simulink model "Copy_of_CM13_2024a_MachE_for_UA_HIL"  (R2024a)
settings: Solver=ode1  StartTime=0.0  StopTime=Inf  FixedStep=0.001  RelTol=1e-3  EnableMultiTasking=on
PreLoadFcn:
  | % if ~length(which('cmcmd')), cmenv; end
PostLoadFcn:
  | if any(exist('dsrtsu_mdlpostloadfcn', 'file') ~= 0), dsrtsu_mdlpostloadfcn('Execute', bdroot); end
InitFcn:
  | , if any(exist('rtifpga_mdlclblib', 'file') ~= 0), rtifpga_mdlclblib('Init', bdroot); end,
  | , if any(exist('dsmpb_private', 'file') ~= 0), dsmpb_private('dsmpb_mdlclblib', 'Init', bdroot); end,
undefined symbols (not defined in the file or in its folder): AccelCmd, ActTqLF_Nm_, ActTqLR_Nm_, ActTqRF_Nm_, ActTqRR_Nm_, BattChargeLimitMaxPwr, BattChargeLimitSocBpts, BattChargeLimitTbl, BattChrgCapcty, BattDischargeLimitSocBpts, BattDischargeLimitTbl, BattDischargeMaxPwr, BattNumCellsParallel, BattNumCellsSeries, BattOpenVoltCapBpts, BattOpenVoltTbl, BattResistSocBpts, BattResistTbl, BattResistTempBpts, BrakeMaxPrs, BrakeMaxTrq, ChassisDistCg2FrontAxle, ChassisDistCg2RearAxle, ChassisVehMass, CltchCmd, CoastDown, DecelCmd, DiffRatio, DiscIntNeverNeededParam, EnvGravCnst, EnvPrs, EnvTemp, FuelSpecificGrav, GearCmd, h, InitStates, lgSw, limitedMCT, MCT, MtrEffSpdBpts, MtrEffTbl, MtrEffTrqBpts, MtrPwrMax, MtrTrqMax, planned_speed, planned_time, pMCT, RealSimPara, ref_speed, Ref_speed, ref_time, Ref_time, rticanmm_blockfcn, rticanmm_initfcn, SteeringCmd, SupvsryCtrlRegenBrkCutOffTbl, SupvsryCtrlRegenSpdBpts, TestScnrioCycleNum, US06, VEH
libraries: simulink x264, VSIGenLib x262, etargetslib x201, dsmpblib x161, CarMaker4SL x142, rtimmsu_dsrtlib x32, vehdynlibtire x24, autolibshared x19, vehdynlibsuspension x14, vehdynlibtirecommon x14, autolibutils x10, VsrLibWheel x8
(part 13 of 47)

== system Copy_of_CM13_2024a_MachE_for_UA_HIL/CarMaker/IPG Vehicle/Actuation and Outputs/MOOG Brake Actuator ==
  Brake Pedal command [%] : Inport
  " CAN Settings" : Subsystem
  BrakePedal Target Position Manual Bypass : Constant  Value=0
  BrakePedal TargetPosition Bypass Enable : Constant  Value=0
  Bus Selector : BusSelector  OutputSignals=ControlWord,TargetPositionFinal_cnt
  ControlWord bypass Enable : Constant  Value=0
  ControlWord bypass Override value : Constant  Value=0
  Data Type Conversion : DataTypeConversion  SaturateOnIntegerOverflow=off  RndMeth=Floor
  Data Type Conversion1 : DataTypeConversion  SaturateOnIntegerOverflow=off  RndMeth=Floor
  Data Type Conversion2 : DataTypeConversion  SaturateOnIntegerOverflow=off  RndMeth=Floor
  Gain : Gain
  Gain1 : Gain
  MOOG Interface : Subsystem
  RPDO3\ControlWord0\ISignal Value\ControlWord0 Value [BrakeAct_Config\Simulated ECUs\CANOpen_MOOG_02\Controller\TX\PDUs] : dsmpblib/Data Outport  Priority=-10000
      settings: SourceProductName=dSPACE Model Interface Package for Simulink (MIPS)
  RPDO3\ModesOfOperation\ISignal Value\ModesOfOperation Value [BrakeAct_Config\Simulated ECUs\CANOpen_MOOG_02\Controller\TX\PDUs] : dsmpblib/Data Outport  Priority=-10000
      settings: SourceProductName=dSPACE Model Interface Package for Simulink (MIPS)
  RPDO3\TargetPosition\ISignal Value\TargetPosition Value [BrakeAct_Config\Simulated ECUs\CANOpen_MOOG_02\Controller\TX\PDUs] : dsmpblib/Data Outport  Priority=-10000
      settings: SourceProductName=dSPACE Model Interface Package for Simulink (MIPS)
  Rate Limiter : RateLimiter  RisingSlewLimit=50  FallingSlewLimit=-50  SampleTimeMode=inherited
  Sine Wave : Sin  Amplitude=50  Bias=50  SampleTime=0
  Switch : Switch  Criteria=u2 > Threshold  SaturateOnIntegerOverflow=off  InputSameDT=off
  Switch1 : Switch  Criteria=u2 > Threshold  SaturateOnIntegerOverflow=off  InputSameDT=off
  Switch2 : Switch  Criteria=u2 > Threshold  SaturateOnIntegerOverflow=off  InputSameDT=off
  TPDO3\ActualPosition\ISignal Value\ActualPosition Value [BrakeAct_Config\Simulated ECUs\CANOpen_MOOG_02\Controller\RX\PDUs] : dsmpblib/Data Inport  Priority=10000
      settings: SourceProductName=dSPACE Model Interface Package for Simulink (MIPS)
  TPDO3\ModesOfOperationDisplay\ISignal Value\ModesOfOperationDisplay Value [BrakeAct_Config\Simulated ECUs\CANOpen_MOOG_02\Controller\RX\PDUs] : dsmpblib/Data Inport  Priority=10000
      settings: SourceProductName=dSPACE Model Interface Package for Simulink (MIPS)
  TPDO3\StatusWord0\ISignal Value\StatusWord0 Value [BrakeAct_Config\Simulated ECUs\CANOpen_MOOG_02\Controller\RX\PDUs] : dsmpblib/Data Inport  Priority=10000
      settings: SourceProductName=dSPACE Model Interface Package for Simulink (MIPS)
  Terminator : Terminator
  Terminator1 : Terminator
  Terminator2 : Terminator
  constant : Constant
  trace selection : Constant  Value=0
  wires:
  Switch/1 -> Switch2/1
  MOOG Interface/1(Commands) -> Bus Selector/1
  MOOG Interface/2(ActualPosition [pct]) -> Terminator/1  "BrakePedal_ActualPosition_pct"
  Bus Selector/2 -> Data Type Conversion2/1  "<TargetPositionFinal_cnt>"
  MOOG Interface/3(BrakeActuatorReady) -> Terminator1/1  "BrakeActuator_Ready_bool"
  Sine Wave/1 -> Switch/1
  Data Type Conversion2/1 -> RPDO3\TargetPosition\ISignal Value\TargetPosition Value [BrakeAct_Config\Simulated ECUs\CANOpen_MOOG_02\Controller\TX\PDUs]/1, Gain1/1  "TargetPosition_Cnt_Final"
  constant/1 -> Data Type Conversion/1
  BrakePedal TargetPosition Bypass Enable/1 -> Switch2/2
  trace selection/1 -> Switch/2
  TPDO3\ModesOfOperationDisplay\ISignal Value\ModesOfOperationDisplay Value [BrakeAct_Config\Simulated ECUs\CANOpen_MOOG_02\Controller\RX\PDUs]/1 -> MOOG Interface/5(Mode of operation in)  "Modes of operations"
  Data Type Conversion1/1 -> RPDO3\ControlWord0\ISignal Value\ControlWord0 Value [BrakeAct_Config\Simulated ECUs\CANOpen_MOOG_02\Controller\TX\PDUs]/1  "ControlWord_Final"
  Gain/1 -> MOOG Interface/2(TargetPosition [pct])  "BrakePedal_TargetlPosition_pct"
  Switch1/1 -> Data Type Conversion1/1
  TPDO3\ActualPosition\ISignal Value\ActualPosition Value [BrakeAct_Config\Simulated ECUs\CANOpen_MOOG_02\Controller\RX\PDUs]/1 -> MOOG Interface/4(ActualPosition_cnt in)  "ActualPosition_cnt"
  Bus Selector/1 -> Switch1/3  "<ControlWord>"
  ControlWord bypass Override value/1 -> Switch1/1
  TPDO3\StatusWord0\ISignal Value\StatusWord0 Value [BrakeAct_Config\Simulated ECUs\CANOpen_MOOG_02\Controller\RX\PDUs]/1 -> MOOG Interface/3(StatusWord in)  "StatusWord0"
  BrakePedal Target Position Manual Bypass/1 -> Rate Limiter/1
  ControlWord bypass Enable/1 -> Switch1/2
  Brake Pedal command [%]/1 -> Switch2/3
  " CAN Settings"/1(CAN_CommsOK_Flg) -> MOOG Interface/1(CAN_CommsOK_Flg)
  Gain1/1 -> Terminator2/1  "BrakePedal_CmdFinal_pct"
  Rate Limiter/1 -> Switch/3
  Switch2/1 -> Gain/1
  Data Type Conversion/1 -> RPDO3\ModesOfOperation\ISignal Value\ModesOfOperation Value [BrakeAct_Config\Simulated ECUs\CANOpen_MOOG_02\Controller\TX\PDUs]/1

== system Copy_of_CM13_2024a_MachE_for_UA_HIL/CarMaker/IPG Vehicle/Actuation and Outputs/Vehicle Accel Pedal Voltage Output ==
  note: Default value for MachE:
      | APP1_CmdFinal_V: 0.8016
      | APP2_CmdFinal_V: 0.4008
  APP_pct : Inport
  APP1Tbl : Lookup_n-D  NumberOfTableDimensions=1  BreakpointsForDimension1=[0 100]  Table=[16 78.8]  InternalRulePriority=Speed  RndMeth=Simplest
  APP2Tbl : Lookup_n-D  NumberOfTableDimensions=1  BreakpointsForDimension1=[0 100]  Table=[8 39.4]  InternalRulePriority=Speed  RndMeth=Simplest
  AccelPosition Bypass Enable : Constant  Value=0
  AccelPosition Manual Bypass [%] : Constant  Value=0
  Gain : Gain
  Gain1 : Gain
  Gain2 : Gain
  Gain3 : Gain  Gain=1/100
  Gain4 : Gain  Gain=1/100
  Product2 : Product
  Product3 : Product
  Rate Limiter : RateLimiter  RisingSlewLimit=50  FallingSlewLimit=-50  SampleTimeMode=inherited
  Switch2 : Switch  Criteria=u2 > Threshold  SaturateOnIntegerOverflow=off  InputSameDT=off
  TPS Channel 1 : dsmpblib/Data Outport  Priority=-10000
      settings: SourceProductName=dSPACE Model Interface Package for Simulink (MIPS)
  TPS Channel 2 : dsmpblib/Data Outport  Priority=-10000
      settings: SourceProductName=dSPACE Model Interface Package for Simulink (MIPS)
  Terminator2 : Terminator
  VRef : Constant  Value=5.01
  wires:
  Switch2/1 -> APP1Tbl/1, APP2Tbl/1, Gain2/1  "APP_CmdFinal_pct"
  APP_pct/1 -> Switch2/3
  AccelPosition Manual Bypass [%]/1 -> Rate Limiter/1
  AccelPosition Bypass Enable/1 -> Switch2/2
  Gain/1 -> TPS Channel 2/1  "APP2_CmdFinal_V"
  Gain1/1 -> TPS Channel 1/1  "APP1_CmdFinal_V"
  Gain2/1 -> Terminator2/1  "AccelPedal_CmdFinal_pct"
  Rate Limiter/1 -> Switch2/1
  VRef/1 -> Product2/2, Product3/1
  Gain4/1 -> Product3/2
  Product2/1 -> Gain1/1
  APP2Tbl/1 -> Gain4/1
  Gain3/1 -> Product2/1
  Product3/1 -> Gain/1
  APP1Tbl/1 -> Gain3/1

== system Copy_of_CM13_2024a_MachE_for_UA_HIL/CarMaker/IPG Vehicle/Brake/CreateBus Vhcl.Wheel.PT ==
  In : Inport
  BusCreator1 : BusCreator  Inputs=20
  Demux1 : Demux  Outputs=20
      settings: DisplayOption=none
  Out : Outport  VectorParamsAs1DForOutWhenUnconnected=off
  wires:
  Demux1/20 -> BusCreator1/20  "Vhcl Trq_DriveSrc_trg d3"
  Demux1/19 -> BusCreator1/19  "Vhcl Trq_DriveSrc_trg d2"
  Demux1/18 -> BusCreator1/18  "Vhcl Trq_DriveSrc_trg d1"
  Demux1/17 -> BusCreator1/17  "Vhcl Trq_DriveSrc_trg d0"
  Demux1/16 -> BusCreator1/16  "Vhcl Wheel RR WhlBearing"
  Demux1/15 -> BusCreator1/15  "Vhcl Wheel RR Trq_T2W"
  Demux1/14 -> BusCreator1/14  "Vhcl Wheel RR Trq_BrakeReg_trg"
  Demux1/13 -> BusCreator1/13  "Vhcl Wheel RR Trq_Brake"
  Demux1/12 -> BusCreator1/12  "Vhcl Wheel RL WhlBearing"
  Demux1/11 -> BusCreator1/11  "Vhcl Wheel RL Trq_T2W"
  Demux1/10 -> BusCreator1/10  "Vhcl Wheel RL Trq_BrakeReg_trg"
  Demux1/9 -> BusCreator1/9  "Vhcl Wheel RL Trq_Brake"
  Demux1/8 -> BusCreator1/8  "Vhcl Wheel FR WhlBearing"
  Demux1/7 -> BusCreator1/7  "Vhcl Wheel FR Trq_T2W"
  Demux1/6 -> BusCreator1/6  "Vhcl Wheel FR Trq_BrakeReg_trg"
  Demux1/5 -> BusCreator1/5  "Vhcl Wheel FR Trq_Brake"
  Demux1/4 -> BusCreator1/4  "Vhcl Wheel FL WhlBearing"
  Demux1/3 -> BusCreator1/3  "Vhcl Wheel FL Trq_T2W"
  Demux1/2 -> BusCreator1/2  "Vhcl Wheel FL Trq_BrakeReg_trg"
  Demux1/1 -> BusCreator1/1  "Vhcl Wheel FL Trq_Brake"
  BusCreator1/1 -> Out/1
  In/1 -> Demux1/1

== system Copy_of_CM13_2024a_MachE_for_UA_HIL/CarMaker/IPG Vehicle/CarAndTrailer/CarAndTrailerUpd ==
  Sync_In : Inport
  Vhcl.Steering : Inport  Port=2
  Vhcl.Motion : Inport  Port=3
  Vhcl.PoI : Inport  Port=4
  Vhcl.Wheel.FL : Inport  Port=5
  Vhcl.Wheel.FR : Inport  Port=6
  Vhcl.Wheel.RL : Inport  Port=7
  Vhcl.Wheel.RR : Inport  Port=8
  Car.Hitch.FrcTrq : Inport  Port=9
  Vhcl.Fr1A : Inport  Port=10
  CarAndTrailerUpd : S-Function  FunctionName=CM_Sfun  Parameters='CarAndTrUpd'  SFunctionDeploymentMode=off  EnableBusSupport=off
  CreateBus Brake.IF.In : Subsystem
  Sync_Out : Outport  VectorParamsAs1DForOutWhenUnconnected=off
  Brake.IF.In : Outport  Port=2  VectorParamsAs1DForOutWhenUnconnected=off
  wires:
  Vhcl.Fr1A/1 -> CarAndTrailerUpd/10  "user vehicle only"
  Vhcl.Steering/1 -> CarAndTrailerUpd/2
  Vhcl.Motion/1 -> CarAndTrailerUpd/3
  Vhcl.PoI/1 -> CarAndTrailerUpd/4
  Vhcl.Wheel.FL/1 -> CarAndTrailerUpd/5
  Vhcl.Wheel.FR/1 -> CarAndTrailerUpd/6
  Car.Hitch.FrcTrq/1 -> CarAndTrailerUpd/9
  Vhcl.Wheel.RR/1 -> CarAndTrailerUpd/8
  Vhcl.Wheel.RL/1 -> CarAndTrailerUpd/7
  CarAndTrailerUpd/2 -> CreateBus Brake.IF.In/1(In)
  CreateBus Brake.IF.In/1(Out) -> Brake.IF.In/1
  CarAndTrailerUpd/1 -> Sync_Out/1
  Sync_In/1 -> CarAndTrailerUpd/1

== system Copy_of_CM13_2024a_MachE_for_UA_HIL/CarMaker/IPG Vehicle/CarAndTrailer/Forces ==
  Sync_In : Inport
  TireFL_In : Inport  Port=2
  TireFR_In : Inport  Port=3
  TireRL_In : Inport  Port=4
  TireRR_In : Inport  Port=5
  lSpring : Inport  Port=6
  vDamp : Inport  Port=7
  lStabi : Inport  Port=8
  lBuf : Inport  Port=9
  External Suspension Forces : Subsystem
  Suspension Forces : Subsystem
  Tires : Subsystem
  Vehicle Forces : Subsystem
  Sync_Out : Outport  VectorParamsAs1DForOutWhenUnconnected=off
  Car.Virtual : Outport  Port=2  VectorParamsAs1DForOutWhenUnconnected=off
  Car.Aero : Outport  Port=3  VectorParamsAs1DForOutWhenUnconnected=off
  Car.Load : Outport  Port=4  VectorParamsAs1DForOutWhenUnconnected=off
  TireFL_Out : Outport  Port=5  VectorParamsAs1DForOutWhenUnconnected=off
  TireFR_Out : Outport  Port=6  VectorParamsAs1DForOutWhenUnconnected=off
  TireRL_Out : Outport  Port=7  VectorParamsAs1DForOutWhenUnconnected=off
  TireRR_Out : Outport  Port=8  VectorParamsAs1DForOutWhenUnconnected=off
  FSpring_ext : Outport  Port=9  VectorParamsAs1DForOutWhenUnconnected=off
  FDamp_ext : Outport  Port=10  VectorParamsAs1DForOutWhenUnconnected=off
  FStabi_ext : Outport  Port=11  VectorParamsAs1DForOutWhenUnconnected=off
  FBuf_ext : Outport  Port=12  VectorParamsAs1DForOutWhenUnconnected=off
  wires:
  lBuf/1 -> External Suspension Forces/5(lBuf), Suspension Forces/5(lBuf)
  lStabi/1 -> External Suspension Forces/4(lStabi), Suspension Forces/4(lStabi)
  vDamp/1 -> External Suspension Forces/3(vDamp), Suspension Forces/3(vDamp)
  Tires/4(TireRR_Out) -> TireRR_Out/1
  Tires/3(TireRL_Out) -> TireRL_Out/1
  Tires/2(TireFR_Out) -> TireFR_Out/1
  Tires/1(TireFL_Out) -> TireFL_Out/1
  TireRR_In/1 -> Tires/5(TireRR_In)
  TireRL_In/1 -> Tires/4(TireRL_In)
  TireFR_In/1 -> Tires/3(TireFR_In)
  TireFL_In/1 -> Tires/2(TireFL_In)
  External Suspension Forces/4(FBuf_ext) -> FBuf_ext/1
  Sync_In/1 -> External Suspension Forces/1(Sync_In), Tires/1(Sync_In), Vehicle Forces/1(Sync_In)
  Vehicle Forces/1(Sync_Out) -> Suspension Forces/1(Sync_In)
  Vehicle Forces/2(Car.Virtual) -> Car.Virtual/1
  Vehicle Forces/3(Car.Aero) -> Car.Aero/1
  Vehicle Forces/4(Car.Load) -> Car.Load/1
  lSpring/1 -> External Suspension Forces/2(lSpring), Suspension Forces/2(lSpring)
  External Suspension Forces/2(FDamp_ext) -> FDamp_ext/1
  External Suspension Forces/3(FStabi_ext) -> FStabi_ext/1
  External Suspension Forces/1(FSpring_ext) -> FSpring_ext/1
  Suspension Forces/1(Sync_Out) -> Sync_Out/1

== system Copy_of_CM13_2024a_MachE_for_UA_HIL/CarMaker/IPG Vehicle/CarAndTrailer/Kinematics ==
  Sync_In : Inport
  Steer.IF : Inport  Port=2
  Kinematics : S-Function  FunctionName=CM_Sfun  Parameters='Kinematics'  SFunctionDeploymentMode=off  EnableBusSupport=off
  Sync_Out : Outport  VectorParamsAs1DForOutWhenUnconnected=off
  TireFL_In : Outport  Port=2  VectorParamsAs1DForOutWhenUnconnected=off
  TireFR_In : Outport  Port=3  VectorParamsAs1DForOutWhenUnconnected=off
  TireRL_In : Outport  Port=4  VectorParamsAs1DForOutWhenUnconnected=off
  TireRR_In : Outport  Port=5  VectorParamsAs1DForOutWhenUnconnected=off
  lSpring : Outport  Port=6  VectorParamsAs1DForOutWhenUnconnected=off
  vDamp : Outport  Port=7  VectorParamsAs1DForOutWhenUnconnected=off
  lStabi : Outport  Port=8  VectorParamsAs1DForOutWhenUnconnected=off
  lBuf : Outport  Port=9  VectorParamsAs1DForOutWhenUnconnected=off
  wires:
  Kinematics/9 -> lBuf/1
  Kinematics/8 -> lStabi/1
  Kinematics/2 -> TireFL_In/1
  Kinematics/3 -> TireFR_In/1
  Kinematics/4 -> TireRL_In/1
  Kinematics/5 -> TireRR_In/1
  Kinematics/6 -> lSpring/1
  Kinematics/7 -> vDamp/1
  Sync_In/1 -> Kinematics/1
  Kinematics/1 -> Sync_Out/1
  Steer.IF/1 -> Kinematics/2

== system Copy_of_CM13_2024a_MachE_for_UA_HIL/CarMaker/IPG Vehicle/CarAndTrailer/Kinetics ==
  Sync_In : Inport
  Car.Virtual : Inport  Port=2
  Car.Aero : Inport  Port=3
  Car.Load : Inport  Port=4
  TireFL.Out : Inport  Port=5
  TireFR.Out : Inport  Port=6
  TireRL.Out : Inport  Port=7
  TireRR.Out : Inport  Port=8
  FSpring_ext : Inport  Port=9
  FDamp_ext : Inport  Port=10
  FStabi_ext : Inport  Port=11
  FBuf_ext : Inport  Port=12
  Bus Creator : BusCreator  Inputs=4
  Bus Creator1 : BusCreator  Inputs=12
  Bus Creator2 : BusCreator  Inputs=6
  Bus Creator3 : BusCreator  Inputs=6
  Bus Creator4 : BusCreator  Inputs=4
  Demux : Demux  Outputs=12
      settings: DisplayOption=none
  Demux1 : Demux  Outputs=6
      settings: DisplayOption=none
  Demux2 : Demux  Outputs=6
      settings: DisplayOption=none
  Demux3 : Demux
      settings: DisplayOption=none
  Demux4 : Demux
      settings: DisplayOption=none
  Kinetics : S-Function  FunctionName=CM_Sfun  Parameters='Kinetics'  SFunctionDeploymentMode=off  EnableBusSupport=off
  Sync_Out : Outport  VectorParamsAs1DForOutWhenUnconnected=off
  Trailer.Load : Outport  Port=2  VectorParamsAs1DForOutWhenUnconnected=off
  Car.Hitch : Outport  Port=3  VectorParamsAs1DForOutWhenUnconnected=off
  Car.Fr1 : Outport  Port=4  VectorParamsAs1DForOutWhenUnconnected=off
  Car.Trq_T2W : Outport  Port=5  VectorParamsAs1DForOutWhenUnconnected=off
  WheelCarrier.Misc : Outport  Port=6  VectorParamsAs1DForOutWhenUnconnected=off
  wires:
  FBuf_ext/1 -> Kinetics/12
  Sync_In/1 -> Kinetics/1
  Kinetics/1 -> Sync_Out/1
  Car.Aero/1 -> Kinetics/3
  Car.Virtual/1 -> Kinetics/2
  Bus Creator1/1 -> Trailer.Load/1
  Demux/1 -> Bus Creator1/1  "Trailer Load_0 mass"
  Demux/2 -> Bus Creator1/2  "Trailer Load_0 tx"
  Demux/3 -> Bus Creator1/3  "Trailer Load_0 ty"
  Demux/4 -> Bus Creator1/4  "Trailer Load_0 tz"
  Kinetics/2 -> Demux/1
  Demux/5 -> Bus Creator1/5  "Trailer Load_1 mass"
  Demux/6 -> Bus Creator1/6  "Trailer Load_1 tx"
  Demux/7 -> Bus Creator1/7  "Trailer Load_1 ty"
  Demux/8 -> Bus Creator1/8  "Trailer Load_1 tz"
  Demux/9 -> Bus Creator1/9  "Trailer Load_2 mass"
  Demux/10 -> Bus Creator1/10  "Trailer Load_2 tx"
  Demux/11 -> Bus Creator1/11  "Trailer Load_2 ty"
  Demux/12 -> Bus Creator1/12  "Trailer Load_2 tz"
  Demux1/1 -> Bus Creator2/1  "Car Hitch tx"
  Demux1/2 -> Bus Creator2/2  "Car Hitch ty"
  Demux1/3 -> Bus Creator2/3  "Car Hitch tz"
  Demux1/4 -> Bus Creator2/4  "Car Hitch vx"
  Demux1/5 -> Bus Creator2/5  "Car Hitch vy"
  Demux1/6 -> Bus Creator2/6  "Car Hitch vz"
  Kinetics/3 -> Demux1/1
  Bus Creator2/1 -> Car.Hitch/1
  Demux2/1 -> Bus Creator3/1  "Car Fr1 rx"
  Demux2/2 -> Bus Creator3/2  "Car Fr1 ry"
  Demux2/3 -> Bus Creator3/3  "Car Fr1 rz"
  Demux2/4 -> Bus Creator3/4  "Car Fr1 rvx"
  Demux2/5 -> Bus Creator3/5  "Car Fr1 rvy"
  Demux2/6 -> Bus Creator3/6  "Car Fr1 rvz"
  Bus Creator3/1 -> Car.Fr1/1
  Kinetics/4 -> Demux2/1
  Car.Load/1 -> Kinetics/4
  Demux3/1 -> Bus Creator4/1  "car Susp FL GenInert2"
  Demux3/2 -> Bus Creator4/2  "car Susp FR GenInert2"
  Demux3/3 -> Bus Creator4/3  "car Susp FL GenFrc2"
  Demux3/4 -> Bus Creator4/4  "car Susp FR GenFrc2"
  Bus Creator4/1 -> WheelCarrier.Misc/1
  Bus Creator/1 -> Car.Trq_T2W/1
  Demux4/4 -> Bus Creator/4  "Car Trq_T2WRR"
  Demux4/3 -> Bus Creator/3  "Car Trq_T2WRL"
  Demux4/2 -> Bus Creator/2  "Car Trq_T2WFR"
  Demux4/1 -> Bus Creator/1  "Car Trq_T2WFL"
  TireFL.Out/1 -> Kinetics/5
  TireFR.Out/1 -> Kinetics/6
  TireRL.Out/1 -> Kinetics/7
  TireRR.Out/1 -> Kinetics/8
  FSpring_ext/1 -> Kinetics/9
  FDamp_ext/1 -> Kinetics/10
  FStabi_ext/1 -> Kinetics/11
  Kinetics/6 -> Demux3/1
  Kinetics/5 -> Demux4/1

== system Copy_of_CM13_2024a_MachE_for_UA_HIL/CarMaker/IPG Vehicle/CarAndTrailer/Steering ==
  note: When replacing the entire steering system,
      | be sure to disable the IPG steering model by using the steering
      | model 'Model Manager off' in the vehicle GUI.
  Sync_In : Inport
  VhclCtrl.Steering : Inport  Port=2
  Bus Creator1 : BusCreator  Inputs=16
  Bus Creator2 : BusCreator  Inputs=5
  Demux : Demux  Outputs=21
      settings: DisplayOption=none
  Steering : S-Function  FunctionName=CM_Sfun  Parameters='Steering'  SFunctionDeploymentMode=off  EnableBusSupport=off
  Terminator : Terminator
  Sync_Out : Outport  VectorParamsAs1DForOutWhenUnconnected=off
  Steer.IF : Outport  Port=2  VectorParamsAs1DForOutWhenUnconnected=off
  wires:
  Demux/21 -> Bus Creator2/5  "Steering IF R Inert"
  Demux/20 -> Bus Creator2/4  "Steering IF R Frc"
  Demux/19 -> Bus Creator2/3  "Steering IF L Inert"
  Demux/18 -> Bus Creator2/2  "Steering IF L Frc"
  Demux/17 -> Bus Creator2/1  "Steering IF SteerByTrq"
  Demux/16 -> Bus Creator1/16  "Steering IF R iSteer2q"
  Demux/15 -> Bus Creator1/15  "Steering IF R qpp"
  Demux/14 -> Bus Creator1/14  "Steering IF R qp"
  Demux/13 -> Bus Creator1/13  "Steering IF R q"
  Demux/12 -> Bus Creator1/12  "Steering IF L iSteer2q"
  Demux/11 -> Bus Creator1/11  "Steering IF L qpp"
  Demux/10 -> Bus Creator1/10  "Steering IF L qp"
  Demux/9 -> Bus Creator1/9  "Steering IF L q"
  Demux/8 -> Bus Creator1/8  "Steering IF AssistTrqPin"
  Demux/7 -> Bus Creator1/7  "Steering IF AssistTrqCol"
  Demux/6 -> Bus Creator1/6  "Steering IF AssistFrc"
  Demux/5 -> Bus Creator1/5  "Steering IF TrqStatic"
  Demux/4 -> Bus Creator1/4  "Steering IF Trq"
  Demux/3 -> Bus Creator1/3  "Steering IF AngAcc"
  Demux/2 -> Bus Creator1/2  "Steering IF AngVel"
  Demux/1 -> Bus Creator1/1  "Steering IF Ang"
  Bus Creator1/1 -> Steer.IF/1
  Steering/2 -> Demux/1
  Bus Creator2/1 -> Terminator/1  "Steer IF (in)"
  VhclCtrl.Steering/1 -> Steering/2
  Steering/1 -> Sync_Out/1
  Sync_In/1 -> Steering/1

== system Copy_of_CM13_2024a_MachE_for_UA_HIL/CarMaker/IPG Vehicle/CarAndTrailer/Trailer ==
  Sync_In : Inport
  Trailer.Load : Inport  Port=2
  Car.Hitch : Inport  Port=3
  Car.Fr1 : Inport  Port=4
  Car.Trq_T2W : Inport  Port=5
  WheelCarrier.Misc : Inport  Port=6
  CreateBus Car.Hitch.FrcTrq : Subsystem
  CreateBus Vhcl.Motion : Subsystem
  CreateBus Vhcl.PoI : Subsystem
  CreateBus Vhcl.Steering : Subsystem
  CreateBus Vhcl.Wheel.FL : Subsystem
  CreateBus Vhcl.Wheel.FR : Subsystem
  CreateBus Vhcl.Wheel.RL : Subsystem
  CreateBus Vhcl.Wheel.RR : Subsystem
  Trailer : S-Function  FunctionName=CM_Sfun  Parameters='Trailer'  SFunctionDeploymentMode=off  EnableBusSupport=off
  Sync_Out : Outport  VectorParamsAs1DForOutWhenUnconnected=off
  Vhcl.Steering : Outport  Port=2  VectorParamsAs1DForOutWhenUnconnected=off
  Vhcl.Motion : Outport  Port=3  VectorParamsAs1DForOutWhenUnconnected=off
  Vhcl.PoI : Outport  Port=4  VectorParamsAs1DForOutWhenUnconnected=off
  Vhcl.Wheel.FL : Outport  Port=5  VectorParamsAs1DForOutWhenUnconnected=off
  Vhcl.Wheel.FR : Outport  Port=6  VectorParamsAs1DForOutWhenUnconnected=off
  Vhcl.Wheel.RL : Outport  Port=7  VectorParamsAs1DForOutWhenUnconnected=off
  Vhcl.Wheel.RR : Outport  Port=8  VectorParamsAs1DForOutWhenUnconnected=off
  Car.Hitch.FrcTrq : Outport  Port=9  VectorParamsAs1DForOutWhenUnconnected=off
  wires:
  Trailer/2 -> CreateBus Vhcl.Steering/1(In1)
  CreateBus Vhcl.Steering/1(Out1) -> Vhcl.Steering/1  "Vhcl.Steering"
  Trailer/3 -> CreateBus Vhcl.Motion/1(In1)
  Trailer/4 -> CreateBus Vhcl.PoI/1(In1)
  Trailer/5 -> CreateBus Vhcl.Wheel.FL/1(In1)
  Trailer/6 -> CreateBus Vhcl.Wheel.FR/1(In1)
  Trailer/7 -> CreateBus Vhcl.Wheel.RL/1(In1)
  Trailer/9 -> CreateBus Car.Hitch.FrcTrq/1(In1)
  Trailer/8 -> CreateBus Vhcl.Wheel.RR/1(In1)
  CreateBus Vhcl.Wheel.RR/1(Out1) -> Vhcl.Wheel.RR/1  "Vhcl.Wheel.RR"
  CreateBus Vhcl.Wheel.RL/1(Out1) -> Vhcl.Wheel.RL/1  "Vhcl.Wheel.RL"
  CreateBus Vhcl.Wheel.FR/1(Out1) -> Vhcl.Wheel.FR/1  "Vhcl.Wheel.FR"
  CreateBus Vhcl.Wheel.FL/1(Out1) -> Vhcl.Wheel.FL/1  "Vhcl.Wheel.FL"
  CreateBus Vhcl.PoI/1(Out1) -> Vhcl.PoI/1  "Vhcl.PoI"
  CreateBus Vhcl.Motion/1(Out1) -> Vhcl.Motion/1  "Vhcl.Motion"
  Car.Trq_T2W/1 -> Trailer/5
  WheelCarrier.Misc/1 -> Trailer/6
  CreateBus Car.Hitch.FrcTrq/1(Out1) -> Car.Hitch.FrcTrq/1  "Car.Hitch.FrcTrq"
  Car.Fr1/1 -> Trailer/4
  Car.Hitch/1 -> Trailer/3
  Trailer.Load/1 -> Trailer/2
  Trailer/1 -> Sync_Out/1
  Sync_In/1 -> Trailer/1

== system Copy_of_CM13_2024a_MachE_for_UA_HIL/CarMaker/IPG Vehicle/Driver and Drive Cycle/Automation_Spd_selection ==
  note: Auther@MaxChen
  note: Note: Since all v_vut is assinged to init velocity,
      | we will use this number as the target testrun speed
  note: If CM reach postprocessing,
      | or vehicle has driven more than 150meter, set speed to 0
  note: TODO: This delay need to be larger. Maybe a real-time of 5 seconds
  note: If AEB flag is triggered, set speed to 0
      | If AEB flag is cleared:
      | 	if Master SW is ON, use TestRun File Speed Demond
      | 	else speed is 0
  AEB_IS_Triggered : Inport
  A_M_SW_sig : Inport  Port=2
  0_speed : Constant  Value=0
  Compare To Constant : simulink/Logic and Bit Operations/Compare To Constant  relop===  const=10  OutDataTypeStr=boolean
  Compare To Constant1 : simulink/Logic and Bit Operations/Compare To Constant  relop=>=  const=150  OutDataTypeStr=boolean
  Delay : Delay  DelayLength=5
  OR : Logic  Operator=OR  IconShape=distinctive  AllPortsSameDT=off  OutDataTypeStr=boolean
  Read CM Dict11 : CarMaker4SL/Read CM Dict  xname=Vhcl.Distance  xsync=off  xstime=Continuous
  Read CM Dict7 : CarMaker4SL/Read CM Dict  xname=SC.State  xsync=off  xstime=Continuous
  Read CM Parameter : CarMaker4SL/Read CM Parameter  xfile=Testrun  xkey=DrivMan.Init.Velocity  xnout=1  xdefaults=0  xmuxed=on  xstime=Continuous
      settings: SourceProductName=CarMaker4SL
  Switch : Switch  Criteria=u2 > Threshold  SaturateOnIntegerOverflow=off  InputSameDT=off
  Switch1 : Switch  Criteria=u2 > Threshold  SaturateOnIntegerOverflow=off  InputSameDT=off
  Switch2 : Switch  Criteria=u2 > Threshold  SaturateOnIntegerOverflow=off  InputSameDT=off
  Spd : Outport
  wires:
  AEB_IS_Triggered/1 -> Switch/2
  Switch/1 -> Switch2/3
  A_M_SW_sig/1 -> Delay/1
  0_speed/1 -> Switch1/3, Switch/1, Switch2/1
  Switch1/1 -> Switch/3
  Delay/1 -> Switch1/2
  Read CM Dict7/1 -> Compare To Constant/1  "SC.State"
  Compare To Constant/1 -> OR/2
  Switch2/1 -> Spd/1
  Read CM Parameter/1 -> Switch1/1  "v_vut"
  Read CM Dict11/1 -> Compare To Constant1/1  "Vhcl.Distance"
  Compare To Constant1/1 -> OR/1
  OR/1 -> Switch2/2

== system Copy_of_CM13_2024a_MachE_for_UA_HIL/CarMaker/IPG Vehicle/Driver and Drive Cycle/Driver and PI with FF Control ==
  Vehicle_Spd_kph : Inport
  Vehicle_SpdDmd_kph : Inport  Port=2
  Bus Creator : BusCreator  Inputs=6
  Constant : Constant
  Memory1 : Memory
  Memory2 : Memory
  SpdSat : Saturate  UpperLimit=190  LowerLimit=-5
  Vehicle Speed Controller : Subsystem
  km to miles : Gain  Gain=1/1.609344
  DriverBus : Outport
  wires:
  Vehicle Speed Controller/1(AcceleratorPedalPos) -> Bus Creator/2  "AccelPedalCmd"
  Vehicle_SpdDmd_kph/1 -> Memory1/1
  Constant/1 -> Bus Creator/1  "Drive"
  Vehicle Speed Controller/3(BrakeSwitch) -> Bus Creator/4
  SpdSat/1 -> Vehicle Speed Controller/1(RefSpd), km to miles/1, Bus Creator/5  "RefSpd [km/hr]"
  Vehicle Speed Controller/2(BrakePedalPos) -> Bus Creator/3  "BrakePedalCmd"
  Bus Creator/1 -> DriverBus/1  "DriverBus"
  Vehicle_Spd_kph/1 -> Memory2/1
  km to miles/1 -> Bus Creator/6  "RefSpd [mph]"
  Memory1/1 -> SpdSat/1
  Memory2/1 -> Vehicle Speed Controller/2(VehicleSpeed)

== system Copy_of_CM13_2024a_MachE_for_UA_HIL/CarMaker/IPG Vehicle/Driver and Drive Cycle/Get Cycle Clock Time ==
  Cycle Trigger : Inport
  Add1 : Sum  Inputs=+-
  Clock1 : Clock
  Clock2 : Clock
  Data Type Conversion : DataTypeConversion  OutDataTypeStr=double  SaturateOnIntegerOverflow=off  RndMeth=Floor
  Memory4 : Memory
  Switch : Switch  Criteria=u2 > Threshold  SaturateOnIntegerOverflow=off  InputSameDT=off
  tCycle : Outport
  wires:
  Switch/1 -> Add1/2, Memory4/1
  Clock1/1 -> Add1/1
  Clock2/1 -> Switch/3
  Add1/1 -> tCycle/1  "tCycle"
  Memory4/1 -> Switch/1
  Cycle Trigger/1 -> Data Type Conversion/1
  Data Type Conversion/1 -> Switch/2

== system Copy_of_CM13_2024a_MachE_for_UA_HIL/CarMaker/IPG Vehicle/Driver and Drive Cycle/IDM ==
  note: In IPG, when the ego vehicle slipped side to side, it will ignore the front vehicle as in the path. The <RadarL> "detects nearest point in the path" , thus ego vehilce will no longer consider the front vehilce as "in path" and ACC/IDM will have incorrect output.
      |
      | Second object sensor <Backup> is added, it dectects nearest point, ensuring ego vehicle stopped at close range.
  CM_Time : Inport
  Add1 : Sum
  Add2 : Sum
  Add3 : Sum  Commented=on
  Bus Selector : BusSelector  OutputSignals=NearPnt ds x,NearPnt ds y,NearPnt dv x
  Bus Selector1 : BusSelector  OutputSignals=dtct
  Bus Selector2 : BusSelector  OutputSignals=dtct
  Bus Selector3 : BusSelector  OutputSignals=NearPnt ds x,NearPnt ds y
  Bus Selector4 : BusSelector  Commented=on  OutputSignals=NearPnt ds x,NearPnt ds y,NearPnt dv x
  Bus Selector5 : BusSelector  Commented=on  OutputSignals=dtct
  Bus Selector6 : BusSelector  OutputSignals=Dist,Vrel
  Compare To Constant : simulink/Logic and Bit Operations/Compare To Constant  relop=>=  const=30  OutDataTypeStr=boolean
  Constant : Constant  Value=0
  Constant1 : Constant  Value=99999
  Constant2 : Constant  Value=99999
  Dis2lead_Raw : Scope
  Math Function{,1..3} (4 alike) : Math  Operator=square
  Math Function4 : Math  Commented=on  Operator=square
  Math Function5 : Math  Commented=on  Operator=square
  ObjIndex : Scope
  Object Sensor 1 : CarMaker4SL/Sensors/Object Sensor  xname=RadarS  xstime=Continuous
      settings: SourceProductName=CarMaker4SL
  Object Sensor 2 : CarMaker4SL/Sensors/Object Sensor  xname=RadarL  xstime=Continuous
      settings: SourceProductName=CarMaker4SL
  Object Sensor Object : CarMaker4SL/Sensors/Object Sensor Object  Commented=on  xname=RadarL  ximode=Observed Objects  xstime=Continuous
      settings: SourceProductName=CarMaker4SL
  Object Sensor Object 1 : CarMaker4SL/Sensors/Object Sensor Object  xname=INPORT  ximode=Observed Objects  xstime=Continuous
      settings: SourceProductName=CarMaker4SL
  Object Sensor Object 2 : CarMaker4SL/Sensors/Object Sensor Object  xname=INPORT  ximode=Observed Objects  xstime=Continuous
      settings: SourceProductName=CarMaker4SL
  Radar Sensor : CarMaker4SL/Sensors/Radar Sensor  xname=RadarReal  xstime=Continuous
      settings: SourceProductName=CarMaker4SL
  Radar Sensor Object : CarMaker4SL/Sensors/Radar Sensor Object  xname=INPORT  ximode=Observed Objects  xstime=Continuous
      settings: SourceProductName=CarMaker4SL
  Read CM Dict1 : CarMaker4SL/Read CM Dict  xname=Car.v  xsync=off  xstime=Continuous
  Scope1 : Scope  Commented=on
  Scope2 : Scope  Commented=on
  Scope3 : Scope
  Scope4 : Scope
  Square Root : Sqrt
  Square Root1 : Sqrt
  Square Root2 : Sqrt  Commented=on
  Subsystem : Subsystem
  Switch1 : Switch  Criteria=u2 > Threshold  SaturateOnIntegerOverflow=off  InputSameDT=off
  ego_ref_spd_m/s : Outport
  wires:
  Add1/1 -> Square Root/1
  Bus Selector1/1 -> Subsystem/1(is_detected)  "<dtct>"
  Bus Selector/3 -> Subsystem/4(rel_front_spd_m/s)  "<NearPnt dv x>"
  Object Sensor Object 2/3 -> Bus Selector1/1
  Read CM Dict1/1 -> Subsystem/2(ego_spd_m/s)  "VehSpd"
  Math Function/1 -> Add1/1
  Object Sensor Object 2/5 -> Bus Selector/1
  Math Function1/1 -> Add1/2
  Object Sensor 2/1 -> Object Sensor Object 2/1
  Constant2/1 -> Object Sensor Object 2/2
  Bus Selector/1 -> Math Function/1  "<NearPnt ds x>"
  Bus Selector/2 -> Math Function1/1  "<NearPnt ds y>"
  Subsystem/1(ego_ref_spd_m/s) -> Switch1/1
  Object Sensor 1/1 -> Object Sensor Object 1/1
  Constant1/1 -> Object Sensor Object 1/2
  Object Sensor Object 1/3 -> Bus Selector2/1
  Bus Selector2/1 -> Subsystem/5(backup_detected)  "<dtct>"
  CM_Time/1 -> [CM_Time]
  Compare To Constant/1 -> Switch1/2
  Constant/1 -> Switch1/3
  Switch1/1 -> ego_ref_spd_m/s/1
  [CM_Time] -> Compare To Constant/1
  Object Sensor Object 1/5 -> Bus Selector3/1
  Math Function3/1 -> Add2/2
  Math Function2/1 -> Add2/1
  Add2/1 -> Square Root1/1
  Bus Selector3/1 -> Math Function2/1  "<NearPnt ds x>"
  Bus Selector3/2 -> Math Function3/1  "<NearPnt ds y>"
  Bus Selector4/2 -> Math Function5/1  "<NearPnt ds y>"
  Bus Selector4/1 -> Math Function4/1  "<NearPnt ds x>"
  Object Sensor Object/3 -> Bus Selector5/1
  Object Sensor Object/5 -> Bus Selector4/1
  Square Root2/1 -> Scope1/1
  Bus Selector4/3 -> Scope2/1  "<NearPnt dv x>"
  Add3/1 -> Square Root2/1
  Math Function4/1 -> Add3/1
  Math Function5/1 -> Add3/2
  Square Root1/1 -> Subsystem/6(front_obj_dist_m)
  Square Root/1 -> Subsystem/3(int_veh_dist_m), Dis2lead_Raw/1
  Radar Sensor/1 -> Radar Sensor Object/1
  Radar Sensor Object/2 -> Bus Selector6/1
  Bus Selector6/1 -> Scope3/1  "<Dist>"
  Bus Selector6/2 -> Scope4/1  "<Vrel>"
  Object Sensor Object 2/1 -> ObjIndex/1

== system Copy_of_CM13_2024a_MachE_for_UA_HIL/CarMaker/IPG Vehicle/Mach-E CAN BM/Subsystem ==
  note: softRCM ECU
  Bus Creator : BusCreator  Inputs=5
  Logic : Subsystem
  Noise Generators : Subsystem  Commented=on
  Read CM Dict : CarMaker4SL/Read CM Dict  xname=Car.RollVel  xsync=off  xstime=Continuous
  Read CM Dict1 : CarMaker4SL/Read CM Dict  xname=Car.YawRate  xsync=off  xstime=Continuous
  Read CM Dict2 : CarMaker4SL/Read CM Dict  xname=Car.ax  xsync=off  xstime=Continuous
  Read CM Dict3 : CarMaker4SL/Read CM Dict  xname=Car.ay  xsync=off  xstime=Continuous
  Read CM Dict4 : CarMaker4SL/Read CM Dict  xname=Car.az  xsync=off  xstime=Continuous
  AccelYaw_out : Outport
  wires:
  Logic/1(Out1) -> AccelYaw_out/1
  Bus Creator/1 -> Logic/1(In1)
  Read CM Dict4/1 -> Bus Creator/5  "a_z_Vehicle_CoG_withG[m|s2]"
  Read CM Dict3/1 -> Bus Creator/4  "a_y_Vehicle_CoG_withG[m|s2]"
  Read CM Dict2/1 -> Bus Creator/3  "a_x_Vehicle_CoG_withG[m|s2]"
  Read CM Dict/1 -> Bus Creator/1  "RollRate_Vehicle_CoG[rad|s]"
  Read CM Dict1/1 -> Bus Creator/2  "YawRate_Vehicle_CoG[rad|s]"

== system Copy_of_CM13_2024a_MachE_for_UA_HIL/CarMaker/IPG Vehicle/Mach-E CAN BM/Subsystem1 ==
  note: softRCM ECU
  Roll : Inport
  Yaw : Inport  Port=2
  A_x : Inport  Port=3
  A_y : Inport  Port=4
  A_z : Inport  Port=5
  Add{,1..4} (5 alike) : Sum
  Bus Creator : BusCreator  Inputs=5
  Logic : Subsystem
  Noise Generators : Subsystem  Commented=on
  Read CM Dict : CarMaker4SL/Read CM Dict  xname=Car.RollVel  xsync=off  xstime=Continuous
  Read CM Dict1 : CarMaker4SL/Read CM Dict  xname=Car.YawRate  xsync=off  xstime=Continuous
  Read CM Dict2 : CarMaker4SL/Read CM Dict  xname=Car.ax  xsync=off  xstime=Continuous
  Read CM Dict3 : CarMaker4SL/Read CM Dict  xname=Car.ay  xsync=off  xstime=Continuous
  Read CM Dict4 : CarMaker4SL/Read CM Dict  xname=Car.az  xsync=off  xstime=Continuous
  AccelYaw_out : Outport
  wires:
  Add/1 -> Bus Creator/5  "a_z_Vehicle_CoG_withG[m|s2]"
  Add2/1 -> Bus Creator/3  "a_x_Vehicle_CoG_withG[m|s2]"
  Add4/1 -> Bus Creator/2  "YawRate_Vehicle_CoG[rad|s]"
  Add1/1 -> Bus Creator/4  "a_y_Vehicle_CoG_withG[m|s2]"
  Add3/1 -> Bus Creator/1  "RollRate_Vehicle_CoG[rad|s]"
  Logic/1(Out1) -> AccelYaw_out/1
  Bus Creator/1 -> Logic/1(In1)
  Read CM Dict4/1 -> Add/1  "a_z_Vehicle_CoG_withG[m|s2]"
  Read CM Dict3/1 -> Add1/1  "a_y_Vehicle_CoG_withG[m|s2]"
  Read CM Dict2/1 -> Add2/1  "a_x_Vehicle_CoG_withG[m|s2]"
  Read CM Dict/1 -> Add3/1  "RollRate_Vehicle_CoG[rad|s]"
  Read CM Dict1/1 -> Add4/1  "YawRate_Vehicle_CoG[rad|s]"
  Yaw/1 -> Add4/2
  A_x/1 -> Add2/2
  A_y/1 -> Add1/2
  Roll/1 -> Add3/2
  A_z/1 -> Add/2

== system Copy_of_CM13_2024a_MachE_for_UA_HIL/CarMaker/IPG Vehicle/MachE CAN/RTICANMM Gateway ==
  Enable : Inport
  DSRT Data Hook1 : rtimmsu_dsrtlib/Data Hook  ControllerName=RCM_ECU  PortID=RTICANMMRCM_ECU  BlockSet=can  blockdata=struct('version','1.0')
  DSRT Data Hook2 : rtimmsu_dsrtlib/Data Hook  ControllerName=RCM_Harness  PortID=RTICANMMRCM_Harness  BlockSet=can  blockdata=struct('version','1.0')
  ModelClose : Subsystem  mask(RTICANMMModelClose){}
  TRC Exclusion : rtimmsu_dsrtlib/TRC Exclusion
  sfcn : S-Function  InitFcn=rticanmm_initfcn(gcb, 'SFCNs')  FunctionName=RTICANMM_GW_RCM_Gateway  SFunctionDeploymentMode=off  EnableBusSupport=off
      mask init:
      | rticanmm_initfcn(gcb, 'SFCNs')
  Bus1TXCounter : Outport  VectorParamsAs1DForOutWhenUnconnected=off
  Bus1RXCounter : Outport  Port=2  VectorParamsAs1DForOutWhenUnconnected=off
  Bus2TXCounter : Outport  Port=3  VectorParamsAs1DForOutWhenUnconnected=off
  Bus2RXCounter : Outport  Port=4  VectorParamsAs1DForOutWhenUnconnected=off
  wires:
  Enable/1 -> sfcn/1
  sfcn/1 -> Bus1TXCounter/1
  sfcn/2 -> Bus1RXCounter/1
  sfcn/3 -> Bus2TXCounter/1
  sfcn/4 -> Bus2RXCounter/1

== system Copy_of_CM13_2024a_MachE_for_UA_HIL/CarMaker/IPG Vehicle/MachE CAN/RTICANMM GeneralSetup ==
  Constant : Constant
  ModelClose : Subsystem  mask(RTICANMMModelClose){}
  TRC Exclusion : rtimmsu_dsrtlib/TRC Exclusion
  Terminator : Terminator
  wires:
  Constant/1 -> Terminator/1

== system Copy_of_CM13_2024a_MachE_for_UA_HIL/CarMaker/IPG Vehicle/MachE CAN/RTICANMM MachE_HS1 ==
  VariationInput : Inport
  Reset : Inport  Port=2
  DSRT Data Hook : rtimmsu_dsrtlib/Data Hook  ControllerName=MachE_HS1  PortID=RTICANMMMachE_HS1  BlockSet=RTICANMM  blockdata=struct('version','1.0')  MMType=ControllerSetup
  ModelClose : Subsystem  mask(RTICANMMModelClose){}
  RTICANMMCHANNEL_TLC : S-Function  FunctionName=rticanmm_tlc_adv  Parameters='DSRT',-1,-1,-1,500,26711143421  SFunctionDeploymentMode=off  EnableBusSupport=off  mask(RTICANMMCHANNEL_TLC){}
  Variation_DTC : DataTypeConversion
  sfcn : S-Function  InitFcn=rticanmm_initfcn(gcb, 'SFCNs')  FunctionName=RTICANMM_SETUP_MachE_HS1  SFunctionDeploymentMode=off  EnableBusSupport=off
      mask init:
      | rticanmm_initfcn(gcb, 'SFCNs')
  wires:
  Reset/1 -> sfcn/2
  VariationInput/1 -> Variation_DTC/1
  Variation_DTC/1 -> sfcn/1

== system Copy_of_CM13_2024a_MachE_for_UA_HIL/CarMaker/IPG Vehicle/MachE CAN/RTICANMM MainBlock ==
  DSRT Data Hook : rtimmsu_dsrtlib/Data Hook  ControllerName=RCM_ECU  PortID=RTICANMMRCM_ECU  BlockSet=RTICANMM  blockdata=struct('version','1.0')  Variant=RCM_ECU  MMType=mainsetup
  ModelClose : Subsystem  mask(RTICANMMModelClose){}
  TRC Exclusion : rtimmsu_dsrtlib/TRC Exclusion
  converter : Subsystem  mask(CANnedyVector2Bus){}
      mask help: Do not change.
      mask Display: disp('Vector to\nBus')
  sfcn : S-Function  InitFcn=rticanmm_initfcn(gcb, 'SFCNs')  FunctionName=RTICANMM_MAIN_RCM_ECU  SFunctionDeploymentMode=off  EnableBusSupport=off
      mask init:
      | rticanmm_initfcn(gcb, 'SFCNs')
  RX_Data : Outport
  wires:
  converter/1(out) -> RX_Data/1
  sfcn/1 -> converter/1(in_1)
  sfcn/2 -> converter/2(in_2)
  sfcn/3 -> converter/3(in_3)
  sfcn/4 -> converter/4(in_4)
  sfcn/5 -> converter/5(in_5)
  sfcn/6 -> converter/6(in_6)
  sfcn/7 -> converter/7(in_7)
  sfcn/8 -> converter/8(in_8)
  sfcn/9 -> converter/9(in_9)
  sfcn/10 -> converter/10(in_10)
  sfcn/11 -> converter/11(in_11)
  sfcn/12 -> converter/12(in_12)
  sfcn/13 -> converter/13(in_13)
  sfcn/14 -> converter/14(in_14)

== system Copy_of_CM13_2024a_MachE_for_UA_HIL/CarMaker/IPG Vehicle/MachE CAN/RTICANMM MainBlock1 ==
  TXData : Inport
  DSRT Data Hook : rtimmsu_dsrtlib/Data Hook  ControllerName=RCM_Harness  PortID=RTICANMMRCM_Harness  BlockSet=RTICANMM  blockdata=struct('version','1.0')  Variant=RCM_Harness  MMType=mainsetup
  ModelClose : Subsystem  mask(RTICANMMModelClose){}
  TRC Exclusion : rtimmsu_dsrtlib/TRC Exclusion
  TXINselector1 : BusSelector  OutputSignals=Accel_Data.VehLatLongVert_No_Cnt,Accel_Data.VehLatLongVertA_No_Cs,Accel_Data.VehVert2_A_Actl,Accel_Data.VehVertAActl_D_Qf,Accel_Data.VehLong2_A_Actl,Accel_Data.VehLongAActl_D_Qf,Accel_Data.VehLat2_A_Actl,Accel_Data.VehLatAActl_D_Qf,Yaw_Data.VehYawWActl_D_Qf,Yaw_Data.VehRolWActl_D_Qf,Yaw_Data.VehRollYaw_No_Cnt,Yaw_Data.VehRollYawW_No_Cs,Yaw_Data.VehYaw_W_Actl,Yaw_Data.VehRol_W_Actl
  converter : Subsystem  mask(CANnedyVector2Bus){}
      mask help: Do not change.
      mask Display: disp('Vector to\nBus')
  sfcn : S-Function  InitFcn=rticanmm_initfcn(gcb, 'SFCNs')  FunctionName=RTICANMM_MAIN_RCM_Harness  SFunctionDeploymentMode=off  EnableBusSupport=off
      mask init:
      | rticanmm_initfcn(gcb, 'SFCNs')
  RX_Data : Outport
  wires:
  TXData/1 -> TXINselector1/1
  TXINselector1/1 -> sfcn/1  "<VehLatLongVert_No_Cnt>"
  TXINselector1/2 -> sfcn/2  "<VehLatLongVertA_No_Cs>"
  TXINselector1/3 -> sfcn/3  "<VehVert2_A_Actl>"
  TXINselector1/4 -> sfcn/4  "<VehVertAActl_D_Qf>"
  TXINselector1/5 -> sfcn/5  "<VehLong2_A_Actl>"
  TXINselector1/6 -> sfcn/6  "<VehLongAActl_D_Qf>"
  TXINselector1/7 -> sfcn/7  "<VehLat2_A_Actl>"
  TXINselector1/8 -> sfcn/8  "<VehLatAActl_D_Qf>"
  TXINselector1/9 -> sfcn/9  "<VehYawWActl_D_Qf>"
  TXINselector1/10 -> sfcn/10  "<VehRolWActl_D_Qf>"
  TXINselector1/11 -> sfcn/11  "<VehRollYaw_No_Cnt>"
  TXINselector1/12 -> sfcn/12  "<VehRollYawW_No_Cs>"
  TXINselector1/13 -> sfcn/13  "<VehYaw_W_Actl>"
  TXINselector1/14 -> sfcn/14  "<VehRol_W_Actl>"
  converter/1(out) -> RX_Data/1
  sfcn/1 -> converter/1(in_1)

== system Copy_of_CM13_2024a_MachE_for_UA_HIL/CarMaker/IPG Vehicle/MachE CAN/RTICANMM MainBlock2 ==
  TXData : Inport
  DSRT Data Hook : rtimmsu_dsrtlib/Data Hook  ControllerName=MachE_HS1  PortID=RTICANMMMachE_HS1  BlockSet=RTICANMM  blockdata=struct('version','1.0')  Variant=MachE_HS1  MMType=mainsetup
  ModelClose : Subsystem  mask(RTICANMMModelClose){}
  TRC Exclusion : rtimmsu_dsrtlib/TRC Exclusion
  TXINselector1 : BusSelector  OutputSignals=Gear_Shift_by_Wire_3_HS1.TrnGear_D_RqPt
  sfcn : S-Function  InitFcn=rticanmm_initfcn(gcb, 'SFCNs')  FunctionName=RTICANMM_MAIN_MachE_HS1  SFunctionDeploymentMode=off  EnableBusSupport=off
      mask init:
      | rticanmm_initfcn(gcb, 'SFCNs')
  wires:
  TXData/1 -> TXINselector1/1
  TXINselector1/1 -> sfcn/1  "<TrnGear_D_RqPt>"

== system Copy_of_CM13_2024a_MachE_for_UA_HIL/CarMaker/IPG Vehicle/MachE CAN/RTICANMM RCM_ECU ==
  VariationInput : Inport
  Reset : Inport  Port=2
  DSRT Data Hook : rtimmsu_dsrtlib/Data Hook  ControllerName=RCM_ECU  PortID=RTICANMMRCM_ECU  BlockSet=RTICANMM  blockdata=struct('version','1.0')  MMType=ControllerSetup
  ModelClose : Subsystem  mask(RTICANMMModelClose){}
  RTICANMMCHANNEL_TLC : S-Function  FunctionName=rticanmm_tlc_adv  Parameters='DSRT',-1,-1,-1,500,26711143421  SFunctionDeploymentMode=off  EnableBusSupport=off  mask(RTICANMMCHANNEL_TLC){}
  Variation_DTC : DataTypeConversion
  sfcn : S-Function  InitFcn=rticanmm_initfcn(gcb, 'SFCNs')  FunctionName=RTICANMM_SETUP_RCM_ECU  SFunctionDeploymentMode=off  EnableBusSupport=off
      mask init:
      | rticanmm_initfcn(gcb, 'SFCNs')
  wires:
  Reset/1 -> sfcn/2
  VariationInput/1 -> Variation_DTC/1
  Variation_DTC/1 -> sfcn/1

== system Copy_of_CM13_2024a_MachE_for_UA_HIL/CarMaker/IPG Vehicle/MachE CAN/RTICANMM RCM_Harness ==
  VariationInput : Inport
  Reset : Inport  Port=2
  DSRT Data Hook : rtimmsu_dsrtlib/Data Hook  ControllerName=RCM_Harness  PortID=RTICANMMRCM_Harness  BlockSet=RTICANMM  blockdata=struct('version','1.0')  MMType=ControllerSetup
  ModelClose : Subsystem  mask(RTICANMMModelClose){}
  RTICANMMCHANNEL_TLC : S-Function  FunctionName=rticanmm_tlc_adv  Parameters='DSRT',-1,-1,-1,500,26711143421  SFunctionDeploymentMode=off  EnableBusSupport=off  mask(RTICANMMCHANNEL_TLC){}
  Variation_DTC : DataTypeConversion
  sfcn : S-Function  InitFcn=rticanmm_initfcn(gcb, 'SFCNs')  FunctionName=RTICANMM_SETUP_RCM_Harness  SFunctionDeploymentMode=off  EnableBusSupport=off
      mask init:
      | rticanmm_initfcn(gcb, 'SFCNs')
  BUS_STATE : Outport
  STATUS_STUFF_BIT_ERROR : Outport  Port=2
  STATUS_FORM_ERROR : Outport  Port=3
  STATUS_CRC_ERROR : Outport  Port=4
  STATUS_LOST_RX_NUM : Outport  Port=5
  STATUS_REC_RX_NUM : Outport  Port=6
  STATUS_SENT_TX_NUM : Outport  Port=7
  wires:
  Reset/1 -> sfcn/2
  sfcn/1 -> BUS_STATE/1
  sfcn/2 -> STATUS_STUFF_BIT_ERROR/1
  sfcn/3 -> STATUS_FORM_ERROR/1
  sfcn/4 -> STATUS_CRC_ERROR/1
  sfcn/5 -> STATUS_LOST_RX_NUM/1
  sfcn/6 -> STATUS_REC_RX_NUM/1
  sfcn/7 -> STATUS_SENT_TX_NUM/1
  VariationInput/1 -> Variation_DTC/1
  Variation_DTC/1 -> sfcn/1

== system Copy_of_CM13_2024a_MachE_for_UA_HIL/CarMaker/IPG Vehicle/MachE CAN/Subsystem ==
  note: softRCM ECU
  Roll : Inport
  Yaw : Inport  Port=2
  A_x : Inport  Port=3
  A_y : Inport  Port=4
  A_z : Inport  Port=5
  Add{,1..4} (5 alike) : Sum
  Bus Creator : BusCreator  Inputs=5
  Logic : Subsystem
  Mapping : Subsystem
  Noise Generators : Subsystem  Commented=on
  Read CM Dict : CarMaker4SL/Read CM Dict  xname=Car.RollVel  xsync=off  xstime=Continuous
  Read CM Dict1 : CarMaker4SL/Read CM Dict  xname=Car.YawRate  xsync=off  xstime=Continuous
  Read CM Dict2 : CarMaker4SL/Read CM Dict  xname=Car.ax  xsync=off  xstime=Continuous
  Read CM Dict3 : CarMaker4SL/Read CM Dict  xname=Car.ay  xsync=off  xstime=Continuous
  Read CM Dict4 : CarMaker4SL/Read CM Dict  xname=Car.az  xsync=off  xstime=Continuous
  Accel_Data_out : Outport
  Yaw_Data_out : Outport  Port=2
  wires:
  Add/1 -> Bus Creator/5  "a_z_Vehicle_CoG_withG[m|s2]"
  Add2/1 -> Bus Creator/3  "a_x_Vehicle_CoG_withG[m|s2]"
  Add4/1 -> Bus Creator/2  "YawRate_Vehicle_CoG[rad|s]"
  Add1/1 -> Bus Creator/4  "a_y_Vehicle_CoG_withG[m|s2]"
  Add3/1 -> Bus Creator/1  "RollRate_Vehicle_CoG[rad|s]"
  Logic/1(Out1) -> Mapping/1(In1)
  Bus Creator/1 -> Logic/1(In1)
  Read CM Dict4/1 -> Add/1  "a_z_Vehicle_CoG_withG[m|s2]"
  Read CM Dict3/1 -> Add1/1  "a_y_Vehicle_CoG_withG[m|s2]"
  Read CM Dict2/1 -> Add2/1  "a_x_Vehicle_CoG_withG[m|s2]"
  Read CM Dict/1 -> Add3/1  "RollRate_Vehicle_CoG[rad|s]"
  Read CM Dict1/1 -> Add4/1  "YawRate_Vehicle_CoG[rad|s]"
  Mapping/1(Accel_Data_Out) -> Accel_Data_out/1  "MsgSignals"
  Mapping/2(Yaw_Data_Out) -> Yaw_Data_out/1
  Yaw/1 -> Add4/2
  A_x/1 -> Add2/2
  A_y/1 -> Add1/2
  Roll/1 -> Add3/2
  A_z/1 -> Add/2

== system Copy_of_CM13_2024a_MachE_for_UA_HIL/CarMaker/IPG Vehicle/MachE CAN/User2RTICANMM MainBlock1 ==
  "Accel_Data " : Inport
  Yaw : Inport  Port=2
  Accel_Data : Subsystem
  Yaw_Data : Subsystem
  buscreator : BusCreator  Inputs=2
  out : Outport
  wires:
  Accel_Data/1(out) -> buscreator/1  "Accel_Data"
  Yaw_Data/1(out) -> buscreator/2  "Yaw_Data"
  buscreator/1 -> out/1  "CAN"
  "Accel_Data "/1 -> Accel_Data/1(Input)
  Yaw/1 -> Yaw_Data/1(Input)

== system Copy_of_CM13_2024a_MachE_for_UA_HIL/CarMaker/IPG Vehicle/MachE CAN/User2RTICANMM MainBlock2 ==
  Gear_Shift_by_Wire_3_HS1 : Subsystem
  buscreator : BusCreator  Inputs=1
  out : Outport
  wires:
  Gear_Shift_by_Wire_3_HS1/1(out) -> buscreator/1  "Gear_Shift_by_Wire_3_HS1"
  buscreator/1 -> out/1  "CAN"

== system Copy_of_CM13_2024a_MachE_for_UA_HIL/CarMaker/IPG Vehicle/Rototest and ORNL Interface/DummyPT ==
  WhlSpeedIn : Inport
  APPToTorque : Lookup_n-D  NumberOfTableDimensions=1  BreakpointsForDimension1=[0 100]  Table=[0 184]  InternalRulePriority=Speed  RndMeth=Simplest
  APPToTorque1 : Lookup_n-D  NumberOfTableDimensions=1  BreakpointsForDimension1=[0 100]  Table=[0 184]  InternalRulePriority=Speed  RndMeth=Simplest
  APP_pct : Constant  Value=0
  BPP_pct : Constant  Value=0
  FDR : Gain  Gain=3.18
  Flip : Gain  Gain=-1
  Gear : Product
  Memory : Memory
  NissanTrans : Lookup_n-D  NumberOfTableDimensions=1  BreakpointsForDimension1=[0 5 10 15 25 34 45 55]  Table=[5.25 3.03 1.95 1.46 1.22 1.00 0.81 0.67]  ExtrapMethod=Clip  InternalRulePriority=Speed  RndMeth=Simplest
  Sum : Sum  Inputs=++|
  WheelRadius : Gain  Gain=0.3235
  kph2mph : Gain  Gain=0.621
  mps2kph : Gain  Gain=3.6
  WheelTorqueOut : Outport
  wires:
  kph2mph/1 -> NissanTrans/1  "Speed_mph"
  APPToTorque/1 -> Sum/1  "APPTorque"
  mps2kph/1 -> kph2mph/1  "Speed_kph"
  BPP_pct/1 -> APPToTorque1/1
  NissanTrans/1 -> Gear/2  "Gear"
  Gear/1 -> FDR/1  "TransTorqueOut"
  APPToTorque1/1 -> Flip/1
  Flip/1 -> Sum/2  "BPPTorque"
  APP_pct/1 -> APPToTorque/1
  Sum/1 -> Gear/1  "TorqueTotal"
  WheelRadius/1 -> mps2kph/1  "Speed_mps"
  FDR/1 -> Memory/1  "WheelTorqueOut"
  WhlSpeedIn/1 -> WheelRadius/1
  Memory/1 -> WheelTorqueOut/1
